simulink model "f16_hifi_euler_vTrim"  (R2020b)
settings: Solver=ode4  StartTime=0.0  StopTime=simTime  FixedStep=stepTime  RelTol=1e-3
undefined symbols (not defined in the file): data, ft, outputs, s
libraries: libAeroLookUpTables x9, aerolibconvert2 x7, lib6DOFUtilityEquations x6, libTFActuatorCalc x5, aerolibtransform2 x1, libEngineAngMomSpecs x1, libAircraftMoISpecs x1, libAircraftWeightandMassSpec x1, libAircraftWingFusalageSpecs x1, libCmdPowConversion x1, libEngineThrustCalc x1, libAtmosphereModel x1
(part 3 of 3)

== system f16_hifi_euler_vTrim/F-16 HiFi Model/Aerodynamic Model/Subsystem/Aerodynamic Forces ==
  note: Wind Axis Forces
  note: Direction Cosine Matrix
  note: Coeffs
  note: Forces
  note: Input Variables
  note: Units
      | Inputs:
      | C_{i}: [ ]
      | qbar: lb/ft^2
      | S: ft^2
      | alpha: deg
      | beta: deg
      | Outputs:
      | F_{i}: lbf
      | M_{i}: lbf*ft
  C_i : Inport
  qbar : Inport  Port=2
  alpha : Inport  Port=3
  beta : Inport  Port=4
  Constant : Constant  Value=S
  Demux : Demux  Outputs=3
  Demux1 : Demux  Outputs=3
  Direction Cosine Matrix Body to Wind : aerolibtransform2/Direction Cosine Matrix Body to Wind
      settings: SourceProductBaseCode=AE
  Gain : Gain  Gain=-1
  Matrix Multiply : Product  Multiplication=Matrix(*)
  Mux : Mux  Inputs=2
  Mux1 : Mux  Inputs=3
  Product : Product  Inputs=3
  Product1 : Product  Inputs=3
  Product2 : Product  Inputs=3
  Fx : Outport  VectorParamsAs1DForOutWhenUnconnected=off
  Fy : Outport  Port=2  VectorParamsAs1DForOutWhenUnconnected=off
  Fz : Outport  Port=3  VectorParamsAs1DForOutWhenUnconnected=off
  D : Outport  Port=4  VectorParamsAs1DForOutWhenUnconnected=off
  C : Outport  Port=5  VectorParamsAs1DForOutWhenUnconnected=off
  L : Outport  Port=6  VectorParamsAs1DForOutWhenUnconnected=off
  wires:
  qbar/1 -> [qbar]
  Constant/1 -> [S]
  Demux/1 -> [Cx]
  Demux/2 -> [Cy]
  Demux/3 -> [Cz]
  [S] -> Product/3
  [qbar] -> Product/2
  [Cz] -> Product/1
  [S] -> Product2/3
  [qbar] -> Product2/2
  [Cx] -> Product2/1
  [Cy] -> Product1/1
  [qbar] -> Product1/2
  [S] -> Product1/3
  Product2/1 -> Fx/1, Mux1/1
  Product1/1 -> Fy/1, Mux1/2
  Product/1 -> Fz/1, Mux1/3
  C_i/1 -> Demux/1
  alpha/1 -> [alpha]
  beta/1 -> [beta]
  [alpha] -> Mux/1
  [beta] -> Mux/2
  Mux/1 -> Direction Cosine Matrix Body to Wind/1
  Direction Cosine Matrix Body to Wind/1 -> Matrix Multiply/1
  Mux1/1 -> Matrix Multiply/2
  Matrix Multiply/1 -> Gain/1
  Gain/1 -> Demux1/1
  Demux1/1 -> D/1
  Demux1/2 -> C/1
  Demux1/3 -> L/1

== system f16_hifi_euler_vTrim/F-16 HiFi Model/Aerodynamic Model/Subsystem/Aerodynamic Moments ==
  note: Moments
  note: Input Variables
  note: Coeffs
  note: Units
      | Inputs:
      | C_{i}: [ ]
      | qbar: lb/ft^2
      | S: ft^2
      | cbar: ft
      | b: ft
      | Outputs:
      | F_{i}: lbf
      | M_{i}: lbf*ft
  C_i : Inport
  qbar : Inport  Port=2
  Constant : Constant  Value=S
  Constant1 : Constant  Value=cbar
  Constant2 : Constant  Value=b
  Demux : Demux  Outputs=3
  Product6 : Product  Inputs=4
  Product7 : Product  Inputs=4
  Product8 : Product  Inputs=4
  Ml : Outport  VectorParamsAs1DForOutWhenUnconnected=off
  Mm : Outport  Port=2  VectorParamsAs1DForOutWhenUnconnected=off
  Mn : Outport  Port=3  VectorParamsAs1DForOutWhenUnconnected=off
  wires:
  [qbar] -> Product7/2
  Constant1/1 -> [cbar]
  [S] -> Product7/3
  [b] -> Product8/4
  [Cm] -> Product7/1
  [Cn] -> Product6/1
  [S] -> Product6/3
  [cbar] -> Product7/4
  Constant2/1 -> [b]
  Constant/1 -> [S]
  [b] -> Product6/4
  [Cl] -> Product8/1
  [qbar] -> Product6/2
  [qbar] -> Product8/2
  Product8/1 -> Ml/1
  Product7/1 -> Mm/1
  qbar/1 -> [qbar]
  [S] -> Product8/3
  Product6/1 -> Mn/1
  C_i/1 -> Demux/1
  Demux/3 -> [Cn]
  Demux/2 -> [Cm]
  Demux/1 -> [Cl]

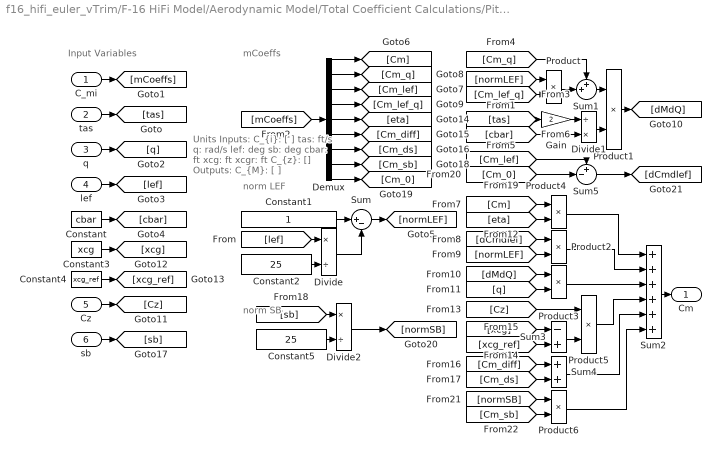
== system f16_hifi_euler_vTrim/F-16 HiFi Model/Aerodynamic Model/Total Coefficient Calculations/Pitch Moment Coefficients ==
  note: norm SB
  note: norm LEF
  note: Input Variables
  note: mCoeffs
  note: Units
      | Inputs:
      | C_{i}: [ ]
      | tas: ft/s
      | q: rad/s
      | lef: deg
      | sb: deg
      | cbar: ft
      | xcg: ft
      | xcgr: ft
      | C_{z}: []
      | Outputs:
      | C_{M}: [ ]
  C_mi : Inport
  tas : Inport  Port=2
  q : Inport  Port=3
  lef : Inport  Port=4
  Cz : Inport  Port=5
  sb : Inport  Port=6
  Constant : Constant  Value=cbar
  Constant1 : Constant
  Constant2 : Constant  Value=25
  Constant3 : Constant  Value=xcg
  Constant4 : Constant  Value=xcg_ref
  Constant5 : Constant  Value=25
  Demux : Demux  Outputs=9
  Divide : Product  Inputs=*/
  Divide1 : Product  Inputs=/*
  Divide2 : Product  Inputs=*/
  Gain : Gain  Gain=2
  Product{,1..6} (7 alike) : Product
  Sum : Sum  Inputs=|+-
  Sum1 : Sum  Inputs=++|
  Sum2 : Sum  Inputs=++++++
  Sum3 : Sum  Inputs=-+
  Sum4 : Sum
  Sum5 : Sum  Inputs=+-|
  Cm : Outport  VectorParamsAs1DForOutWhenUnconnected=off
  wires:
  sb/1 -> [sb]
  [Cm_lef] -> Sum5/1
  [Cm_0] -> Sum5/2
  Product6/1 -> Sum2/6
  [normSB] -> Product6/1
  [Cm_sb] -> Product6/2
  Sum5/1 -> [dCmdlef]
  Divide2/1 -> [normSB]
  [sb] -> Divide2/1
  Constant5/1 -> Divide2/2
  Demux/9 -> [Cm_0]
  Demux/8 -> [Cm_sb]
  Product5/1 -> Sum2/4
  Sum4/1 -> Sum2/5
  [Cm_diff] -> Sum4/1
  [Cm_ds] -> Sum4/2
  Sum3/1 -> Product5/2
  [Cz] -> Product5/1
  [xcg] -> Sum3/1
  [xcg_ref] -> Sum3/2
  Product4/1 -> Sum2/1
  [eta] -> Product4/2
  Demux/5 -> [eta]
  Demux/6 -> [Cm_diff]
  Demux/7 -> [Cm_ds]
  Constant4/1 -> [xcg_ref]
  Constant3/1 -> [xcg]
  Cz/1 -> [Cz]
  tas/1 -> [tas]
  q/1 -> [q]
  Divide/1 -> Sum/2
  C_mi/1 -> [mCoeffs]
  [q] -> Product3/2
  Constant1/1 -> Sum/1
  Constant2/1 -> Divide/2
  Constant/1 -> [cbar]
  lef/1 -> [lef]
  Product/1 -> Sum1/2
  Demux/2 -> [Cm_q]
  [cbar] -> Divide1/2
  [tas] -> Gain/1
  Product3/1 -> Sum2/3
  Sum/1 -> [normLEF]
  [lef] -> Divide/1
  Demux/4 -> [Cm_lef_q]
  Demux/1 -> [Cm]
  [dMdQ] -> Product3/1
  Demux/3 -> [Cm_lef]
  Product1/1 -> [dMdQ]
  [mCoeffs] -> Demux/1
  [normLEF] -> Product/1
  [Cm_lef_q] -> Product/2
  Sum1/1 -> Product1/1
  Gain/1 -> Divide1/1
  Divide1/1 -> Product1/2
  Sum2/1 -> Cm/1
  [Cm_q] -> Sum1/1
  [dCmdlef] -> Product2/1
  [normLEF] -> Product2/2
  [Cm] -> Product4/1
  Product2/1 -> Sum2/2

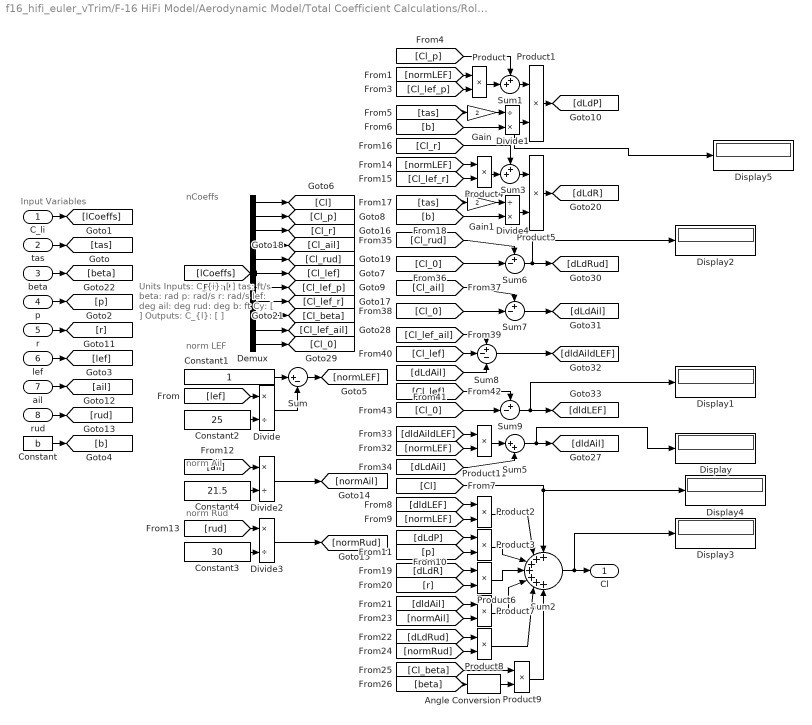
== system f16_hifi_euler_vTrim/F-16 HiFi Model/Aerodynamic Model/Total Coefficient Calculations/Roll Moment Coefficients ==
  note: norm Rud
  note: Input Variables
  note: nCoeffs
  note: norm LEF
  note: norm Ail
  note: Units
      | Inputs:
      | C_{i}: [ ]
      | tas: ft/s
      | beta: rad
      | p: rad/s
      | r: rad/s
      | lef: deg
      | ail: deg
      | rud: deg
      | b: ft
      | Cy: [ ]
      | Outputs:
      | C_{l}: [ ]
  C_li : Inport
  tas : Inport  Port=2
  beta : Inport  Port=3
  p : Inport  Port=4
  r : Inport  Port=5
  lef : Inport  Port=6
  ail : Inport  Port=7
  rud : Inport  Port=8
  Angle Conversion : aerolibconvert2/Angle Conversion  IU=rad  OU=deg
  Constant : Constant  Value=b
  Constant1 : Constant
  Constant2 : Constant  Value=25
  Constant3 : Constant  Value=30
  Constant4 : Constant  Value=21.5
  Demux : Demux  Outputs=11
  Display{,1..5} (6 alike) : Display
  Divide : Product  Inputs=*/
  Divide1 : Product  Inputs=/*
  Divide2 : Product  Inputs=*/
  Divide3 : Product  Inputs=*/
  Divide4 : Product  Inputs=/*
  Gain : Gain  Gain=2
  Gain1 : Gain  Gain=2
  Product{,1..9,11} (11 alike) : Product
  Sum : Sum  Inputs=|+-
  Sum1 : Sum  Inputs=++|
  Sum2 : Sum  Inputs=+++++++
  Sum3 : Sum  Inputs=++|
  Sum5 : Sum  Inputs=|++
  Sum6 : Sum  Inputs=+-|
  Sum7 : Sum  Inputs=+-|
  Sum8 : Sum  Inputs=+--
  Sum9 : Sum  Inputs=+-|
  Cl : Outport  VectorParamsAs1DForOutWhenUnconnected=off
  wires:
  Angle Conversion/1 -> Product9/2
  [beta] -> Angle Conversion/1
  Demux/1 -> [Cl]
  Sum5/1 -> Display/1, [dldAil]
  [normLEF] -> Product2/2
  Product1/1 -> [dLdP]
  tas/1 -> [tas]
  Sum2/1 -> Display3/1, Cl/1
  [dLdRud] -> Product8/1
  [Cl_beta] -> Product9/1
  Demux/3 -> [Cl_r]
  Demux/7 -> [Cl_lef_p]
  [ail] -> Divide2/1
  Product8/1 -> Sum2/6
  Constant4/1 -> Divide2/2
  [normLEF] -> Product4/1
  Constant1/1 -> Sum/1
  Sum1/1 -> Product1/1
  Constant/1 -> [b]
  [normLEF] -> Product11/2
  [Cl] -> Display4/1, Sum2/1
  Sum/1 -> [normLEF]
  [dldAil] -> Product7/1
  Product11/1 -> Sum5/1
  rud/1 -> [rud]
  [Cl_lef_r] -> Product4/2
  [tas] -> Gain1/1
  Demux/4 -> [Cl_ail]
  [dLdP] -> Product3/1
  [p] -> Product3/2
  [dldAildLEF] -> Product11/1
  Divide4/1 -> Product5/2
  [dLdAil] -> Sum5/2
  Sum8/1 -> [dldAildLEF]
  Demux/10 -> [Cl_lef_ail]
  Product5/1 -> [dLdR]
  Product9/1 -> Sum2/7
  C_li/1 -> [lCoeffs]
  [b] -> Divide1/2
  [Cl_lef_p] -> Product/2
  Product/1 -> Sum1/2
  Divide2/1 -> [normAil]
  Demux/9 -> [Cl_beta]
  [lef] -> Divide/1
  [b] -> Divide4/2
  p/1 -> [p]
  [r] -> Product6/2
  [normLEF] -> Product/1
  [rud] -> Divide3/1
  Product3/1 -> Sum2/3
  Gain/1 -> Divide1/1
  Constant2/1 -> Divide/2
  Demux/5 -> [Cl_rud]
  Divide/1 -> Sum/2
  Product7/1 -> Sum2/5
  Sum6/1 -> Display2/1, [dLdRud]
  Demux/2 -> [Cl_p]
  [Cl_p] -> Sum1/1
  Product2/1 -> Sum2/2
  [dLdR] -> Product6/1
  Product6/1 -> Sum2/4
  [tas] -> Gain/1
  [normAil] -> Product7/2
  [Cl_r] -> Sum3/1
  Product4/1 -> Sum3/2
  Divide3/1 -> [normRud]
  ail/1 -> [ail]
  Sum3/1 -> Product5/1
  lef/1 -> [lef]
  Demux/6 -> [Cl_lef]
  Gain1/1 -> Divide4/1
  [Cl_0] -> Sum7/2
  Demux/8 -> [Cl_lef_r]
  [dldLEF] -> Product2/1
  r/1 -> [r]
  beta/1 -> [beta]
  [normRud] -> Product8/2
  Constant3/1 -> Divide3/2
  [lCoeffs] -> Demux/1
  Demux/11 -> [Cl_0]
  [Cl_rud] -> Sum6/1
  [Cl_0] -> Sum6/2
  Sum9/1 -> Display1/1, [dldLEF]
  [Cl_0] -> Sum9/2
  [Cl_lef] -> Sum8/2
  [Cl_ail] -> Sum7/1
  Sum7/1 -> [dLdAil]
  [dLdAil] -> Sum8/3
  [Cl_lef] -> Sum9/1
  [Cl_lef_ail] -> Sum8/1
  Divide1/1 -> Display5/1, Product1/2

== system f16_hifi_euler_vTrim/F-16 HiFi Model/Aerodynamic Model/Total Coefficient Calculations/X-Axis Force Coefficients ==
  note: norm SB
  note: xCoeffs
  note: Input Variables
  note: Units
      | Inputs:
      | C_{i}: [ ]
      | tas: ft/s
      | q: rad/s
      | lef: deg
      | sb: deg
      | cbar: ft
      | Outputs:
      | C_{X}: [ ]
  note: norm LEF
  C_xi : Inport
  tas : Inport  Port=2
  q : Inport  Port=3
  lef : Inport  Port=4
  sb : Inport  Port=5
  Constant : Constant  Value=cbar
  Constant1 : Constant
  Constant2 : Constant  Value=25
  Constant3 : Constant  Value=60
  Demux : Demux  Outputs=6
  Divide : Product  Inputs=*/
  Divide1 : Product  Inputs=/**
  Divide2 : Product  Inputs=*/
  Gain : Gain  Gain=2
  Product{,1..3} (4 alike) : Product
  Sum : Sum  Inputs=|+-
  Sum1 : Sum  Inputs=++|
  Sum2 : Sum  Inputs=++++
  Sum3 : Sum  Inputs=+-|
  Cx : Outport  VectorParamsAs1DForOutWhenUnconnected=off
  wires:
  Product3/1 -> Sum2/4
  [normSB] -> Product3/1
  [Cx_sb] -> Product3/2
  Divide2/1 -> [normSB]
  Constant3/1 -> Divide2/2
  [sb] -> Divide2/1
  Sum3/1 -> [dCxLef]
  [Cx_0] -> Sum3/2
  [Cx_lef] -> Sum3/1
  Demux/6 -> [Cx_0]
  [q] -> Divide1/3
  sb/1 -> [sb]
  Demux/5 -> [Cx_sb]
  Sum2/1 -> Cx/1
  [Cx] -> Sum2/1
  [dXdQ] -> Sum2/3
  Product2/1 -> Sum2/2
  [dCxLef] -> Product2/1
  [normLEF] -> Product2/2
  Product1/1 -> [dXdQ]
  Sum1/1 -> Product1/1
  Divide1/1 -> Product1/2
  [cbar] -> Divide1/2
  Gain/1 -> Divide1/1
  [tas] -> Gain/1
  Product/1 -> Sum1/2
  [Cx_q] -> Sum1/1
  [Cx_lef_q] -> Product/2
  [normLEF] -> Product/1
  Demux/4 -> [Cx_lef_q]
  Demux/3 -> [Cx_lef]
  Demux/2 -> [Cx_q]
  Demux/1 -> [Cx]
  [xCoeffs] -> Demux/1
  Sum/1 -> [normLEF]
  Constant1/1 -> Sum/1
  Divide/1 -> Sum/2
  [lef] -> Divide/1
  Constant2/1 -> Divide/2
  Constant/1 -> [cbar]
  lef/1 -> [lef]
  q/1 -> [q]
  C_xi/1 -> [xCoeffs]
  tas/1 -> [tas]

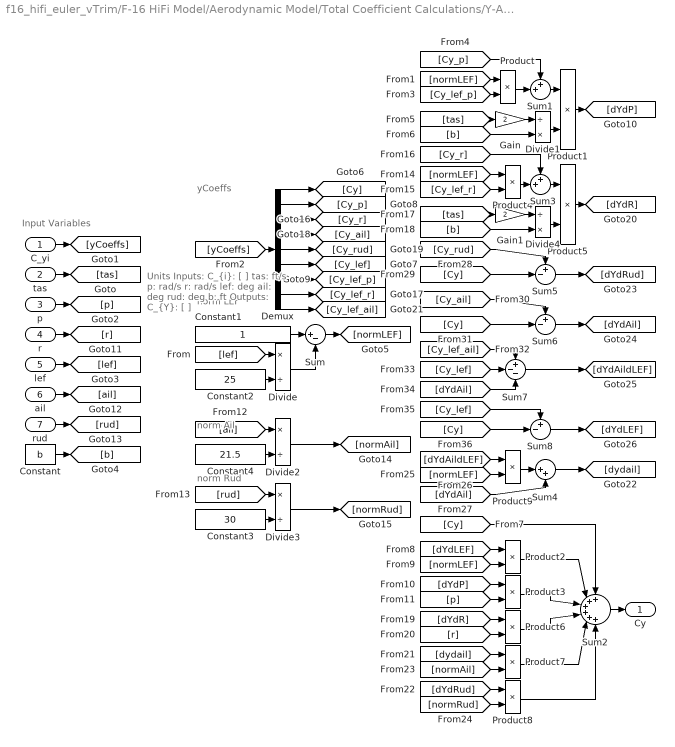
== system f16_hifi_euler_vTrim/F-16 HiFi Model/Aerodynamic Model/Total Coefficient Calculations/Y-Axis Force Coefficients ==
  note: norm Rud
  note: norm Ail
  note: norm LEF
  note: Input Variables
  note: yCoeffs
  note: Units
      | Inputs:
      | C_{i}: [ ]
      | tas: ft/s
      | p: rad/s
      | r: rad/s
      | lef: deg
      | ail: deg
      | rud: deg
      | b: ft
      | Outputs:
      | C_{Y}: [ ]
  C_yi : Inport
  tas : Inport  Port=2
  p : Inport  Port=3
  r : Inport  Port=4
  lef : Inport  Port=5
  ail : Inport  Port=6
  rud : Inport  Port=7
  Constant : Constant  Value=b
  Constant1 : Constant
  Constant2 : Constant  Value=25
  Constant3 : Constant  Value=30
  Constant4 : Constant  Value=21.5
  Demux : Demux  Outputs=9
  Divide : Product  Inputs=*/
  Divide1 : Product  Inputs=/*
  Divide2 : Product  Inputs=*/
  Divide3 : Product  Inputs=*/
  Divide4 : Product  Inputs=/*
  Gain : Gain  Gain=2
  Gain1 : Gain  Gain=2
  Product{,1..9} (10 alike) : Product
  Sum : Sum  Inputs=|+-
  Sum1 : Sum  Inputs=++|
  Sum2 : Sum  Inputs=++++++
  Sum3 : Sum  Inputs=++|
  Sum4 : Sum  Inputs=|++
  Sum5 : Sum  Inputs=+-|
  Sum6 : Sum  Inputs=+-|
  Sum7 : Sum  Inputs=+--
  Sum8 : Sum  Inputs=+-|
  Cy : Outport  VectorParamsAs1DForOutWhenUnconnected=off
  wires:
  [Cy_lef] -> Sum8/1
  [Cy] -> Sum8/2
  Sum8/1 -> [dYdLEF]
  Sum7/1 -> [dYdAildLEF]
  [Cy_lef] -> Sum7/2
  [dYdAil] -> Sum7/3
  [Cy_lef_ail] -> Sum7/1
  [Cy_ail] -> Sum6/1
  Sum6/1 -> [dYdAil]
  [Cy] -> Sum6/2
  Sum5/1 -> [dYdRud]
  [Cy] -> Sum5/2
  [Cy_rud] -> Sum5/1
  Sum4/1 -> [dydail]
  [dYdAil] -> Sum4/2
  Product9/1 -> Sum4/1
  [dYdAildLEF] -> Product9/1
  [normLEF] -> Product9/2
  Demux/9 -> [Cy_lef_ail]
  Product7/1 -> Sum2/5
  Product8/1 -> Sum2/6
  [Cy] -> Sum2/1
  Product2/1 -> Sum2/2
  Product3/1 -> Sum2/3
  Product6/1 -> Sum2/4
  Sum2/1 -> Cy/1
  [dydail] -> Product7/1
  [normAil] -> Product7/2
  [dYdRud] -> Product8/1
  [normRud] -> Product8/2
  [dYdR] -> Product6/1
  [r] -> Product6/2
  Product5/1 -> [dYdR]
  Product4/1 -> Sum3/2
  Gain1/1 -> Divide4/1
  [Cy_r] -> Sum3/1
  [tas] -> Gain1/1
  Sum3/1 -> Product5/1
  [Cy_lef_r] -> Product4/2
  Divide4/1 -> Product5/2
  [normLEF] -> Product4/1
  [b] -> Divide4/2
  Demux/4 -> [Cy_ail]
  Demux/5 -> [Cy_rud]
  Demux/8 -> [Cy_lef_r]
  Demux/3 -> [Cy_r]
  [rud] -> Divide3/1
  Constant3/1 -> Divide3/2
  Divide3/1 -> [normRud]
  Constant4/1 -> Divide2/2
  [ail] -> Divide2/1
  Divide2/1 -> [normAil]
  rud/1 -> [rud]
  ail/1 -> [ail]
  r/1 -> [r]
  Constant1/1 -> Sum/1
  [p] -> Product3/2
  Demux/6 -> [Cy_lef]
  [dYdP] -> Product3/1
  [tas] -> Gain/1
  [Cy_p] -> Sum1/1
  Product/1 -> Sum1/2
  Divide/1 -> Sum/2
  p/1 -> [p]
  Demux/7 -> [Cy_lef_p]
  [lef] -> Divide/1
  tas/1 -> [tas]
  Sum/1 -> [normLEF]
  Constant/1 -> [b]
  [normLEF] -> Product/1
  Product1/1 -> [dYdP]
  [yCoeffs] -> Demux/1
  [b] -> Divide1/2
  C_yi/1 -> [yCoeffs]
  [normLEF] -> Product2/2
  Divide1/1 -> Product1/2
  Gain/1 -> Divide1/1
  Constant2/1 -> Divide/2
  [Cy_lef_p] -> Product/2
  Sum1/1 -> Product1/1
  [dYdLEF] -> Product2/1
  lef/1 -> [lef]
  Demux/1 -> [Cy]
  Demux/2 -> [Cy_p]

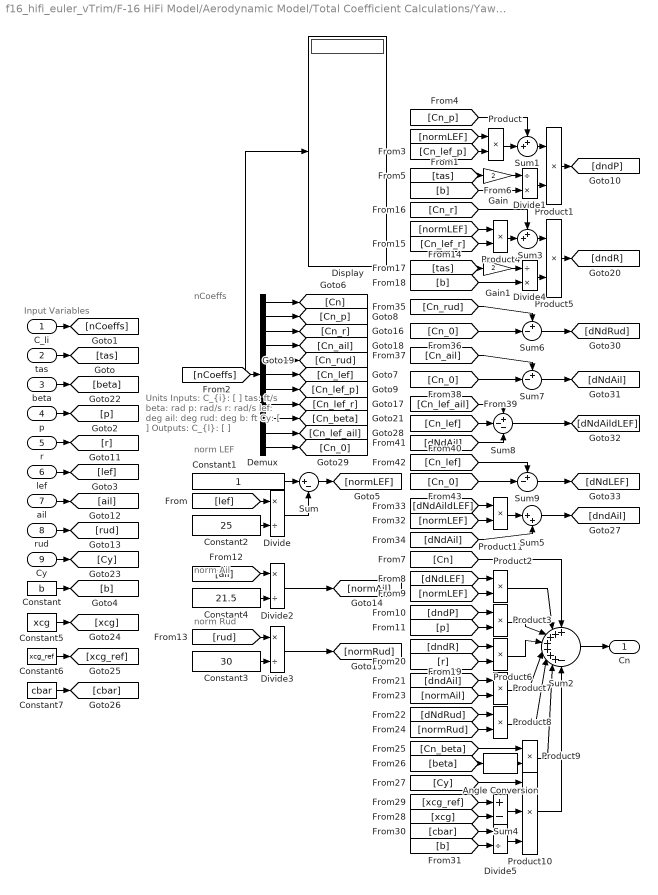
== system f16_hifi_euler_vTrim/F-16 HiFi Model/Aerodynamic Model/Total Coefficient Calculations/Yaw Moment Coefficients ==
  note: norm Rud
  note: norm Ail
  note: norm LEF
  note: Units
      | Inputs:
      | C_{i}: [ ]
      | tas: ft/s
      | beta: rad
      | p: rad/s
      | r: rad/s
      | lef: deg
      | ail: deg
      | rud: deg
      | b: ft
      | Cy: [ ]
      | Outputs:
      | C_{l}: [ ]
  note: nCoeffs
  note: Input Variables
  C_li : Inport
  tas : Inport  Port=2
  beta : Inport  Port=3
  p : Inport  Port=4
  r : Inport  Port=5
  lef : Inport  Port=6
  ail : Inport  Port=7
  rud : Inport  Port=8
  Cy : Inport  Port=9
  Angle Conversion : aerolibconvert2/Angle Conversion  IU=rad  OU=deg
  Constant : Constant  Value=b
  Constant1 : Constant
  Constant2 : Constant  Value=25
  Constant3 : Constant  Value=30
  Constant4 : Constant  Value=21.5
  Constant5 : Constant  Value=xcg
  Constant6 : Constant  Value=xcg_ref
  Constant7 : Constant  Value=cbar
  Demux : Demux  Outputs=11
  Display : Display
  Divide{,2..3,5} (4 alike) : Product  Inputs=*/
  Divide1 : Product  Inputs=/*
  Divide4 : Product  Inputs=/*
  Gain : Gain  Gain=2
  Gain1 : Gain  Gain=2
  Product{,1..9,11} (11 alike) : Product
  Product10 : Product  Inputs=3
  Sum : Sum  Inputs=|+-
  Sum1 : Sum  Inputs=++|
  Sum2 : Sum  Inputs=+++++++-
  Sum3 : Sum  Inputs=++|
  Sum4 : Sum  Inputs=+-
  Sum5 : Sum  Inputs=|++
  Sum6 : Sum  Inputs=+-|
  Sum7 : Sum  Inputs=+-|
  Sum8 : Sum  Inputs=+--
  Sum9 : Sum  Inputs=+-|
  Cn : Outport  VectorParamsAs1DForOutWhenUnconnected=off
  wires:
  Angle Conversion/1 -> Product9/2
  [beta] -> Angle Conversion/1
  [Cn_lef] -> Sum9/1
  [Cn_lef_ail] -> Sum8/1
  [dNdAil] -> Sum8/3
  [Cn_ail] -> Sum7/1
  Sum7/1 -> [dNdAil]
  [Cn_0] -> Sum9/2
  [Cn_lef] -> Sum8/2
  [Cn_0] -> Sum7/2
  [Cn_0] -> Sum6/2
  Sum9/1 -> [dNdLEF]
  [Cn_rud] -> Sum6/1
  Sum8/1 -> [dNdAildLEF]
  Demux/11 -> [Cn_0]
  Demux/10 -> [Cn_lef_ail]
  [dNdAildLEF] -> Product11/1
  Product11/1 -> Sum5/1
  [normLEF] -> Product11/2
  Sum5/1 -> [dndAil]
  [dNdAil] -> Sum5/2
  Product10/1 -> Sum2/8
  [Cy] -> Product10/1
  Divide5/1 -> Product10/3
  Sum4/1 -> Product10/2
  [b] -> Divide5/2
  [cbar] -> Divide5/1
  [xcg] -> Sum4/2
  [xcg_ref] -> Sum4/1
  Constant7/1 -> [cbar]
  Constant5/1 -> [xcg]
  Constant6/1 -> [xcg_ref]
  Cy/1 -> [Cy]
  [Cn_beta] -> Product9/1
  r/1 -> [r]
  Sum/1 -> [normLEF]
  Sum2/1 -> Cn/1
  lef/1 -> [lef]
  Demux/6 -> [Cn_lef]
  rud/1 -> [rud]
  ail/1 -> [ail]
  beta/1 -> [beta]
  [normRud] -> Product8/2
  [Cn_lef_r] -> Product4/2
  Gain1/1 -> Divide4/1
  Constant3/1 -> Divide3/2
  Demux/1 -> [Cn]
  Product6/1 -> Sum2/4
  Demux/5 -> [Cn_rud]
  Product7/1 -> Sum2/5
  Divide3/1 -> [normRud]
  [dndR] -> Product6/1
  Product8/1 -> Sum2/6
  Product4/1 -> Sum3/2
  Demux/8 -> [Cn_lef_r]
  Demux/7 -> [Cn_lef_p]
  Constant4/1 -> Divide2/2
  [Cn_r] -> Sum3/1
  Demux/2 -> [Cn_p]
  Gain/1 -> Divide1/1
  Divide/1 -> Sum/2
  [ail] -> Divide2/1
  [Cn_p] -> Sum1/1
  Product2/1 -> Sum2/2
  [tas] -> Gain/1
  Product3/1 -> Sum2/3
  [p] -> Product3/2
  Sum3/1 -> Product5/1
  Constant1/1 -> Sum/1
  Constant2/1 -> Divide/2
  [normLEF] -> Product4/1
  [dNdRud] -> Product8/1
  [rud] -> Divide3/1
  Demux/4 -> [Cn_ail]
  [b] -> Divide4/2
  [normLEF] -> Product/1
  p/1 -> [p]
  [lef] -> Divide/1
  tas/1 -> [tas]
  Divide2/1 -> [normAil]
  [r] -> Product6/2
  Sum1/1 -> Product1/1
  Product/1 -> Sum1/2
  Divide1/1 -> Product1/2
  Demux/3 -> [Cn_r]
  [Cn] -> Sum2/1
  Constant/1 -> [b]
  Divide4/1 -> Product5/2
  [Cn_lef_p] -> Product/2
  [dNdLEF] -> Product2/1
  [b] -> Divide1/2
  [normAil] -> Product7/2
  [dndP] -> Product3/1
  [dndAil] -> Product7/1
  [tas] -> Gain1/1
  [normLEF] -> Product2/2
  C_li/1 -> [nCoeffs]
  Product9/1 -> Sum2/7
  Demux/9 -> [Cn_beta]
  Product1/1 -> [dndP]
  Product5/1 -> [dndR]
  Sum6/1 -> [dNdRud]
  [nCoeffs] -> Display/1, Demux/1

== system f16_hifi_euler_vTrim/F-16 HiFi Model/Aerodynamic Model/Total Coefficient Calculations/Z-Axis Force Coefficients ==
  note: xCoeffs
  note: Units
      | Inputs:
      | C_{i}: [ ]
      | tas: ft/s
      | q: rad/s
      | lef: deg
      | sb: deg
      | cbar: ft
      | Outputs:
      | C_{X}: [ ]
  note: norm LEF
  note: Input Variables
  note: norm SB
  C_zi : Inport
  tas : Inport  Port=2
  q : Inport  Port=3
  lef : Inport  Port=4
  sb : Inport  Port=5
  Constant : Constant  Value=cbar
  Constant1 : Constant
  Constant2 : Constant  Value=25
  Constant3 : Constant  Value=25
  Demux : Demux  Outputs=6
  Divide : Product  Inputs=*/
  Divide1 : Product  Inputs=/**
  Divide2 : Product  Inputs=*/
  Gain : Gain  Gain=2
  Product{,1..3} (4 alike) : Product
  Sum : Sum  Inputs=|+-
  Sum1 : Sum  Inputs=++|
  Sum2 : Sum  Inputs=++++
  Sum3 : Sum  Inputs=+-|
  Cz : Outport  VectorParamsAs1DForOutWhenUnconnected=off
  wires:
  tas/1 -> [tas]
  Divide/1 -> Sum/2
  Demux/3 -> [Cz_lef]
  Divide2/1 -> [normSB]
  [Cz] -> Sum2/1
  [normLEF] -> Product2/2
  Product1/1 -> [dZdQ]
  Sum1/1 -> Product1/1
  lef/1 -> [lef]
  Product2/1 -> Sum2/2
  Sum/1 -> [normLEF]
  Sum2/1 -> Cz/1
  [tas] -> Gain/1
  Demux/6 -> [Cz_0]
  Gain/1 -> Divide1/1
  [cbar] -> Divide1/2
  [zCoeffs] -> Demux/1
  [Cz_lef] -> Sum3/1
  [q] -> Divide1/3
  Product/1 -> Sum1/2
  Demux/2 -> [Cz_q]
  Constant2/1 -> Divide/2
  C_zi/1 -> [zCoeffs]
  [lef] -> Divide/1
  sb/1 -> [sb]
  Sum3/1 -> [dCzLef]
  Constant1/1 -> Sum/1
  Constant/1 -> [cbar]
  q/1 -> [q]
  Divide1/1 -> Product1/2
  Demux/1 -> [Cz]
  [dCzLef] -> Product2/1
  Demux/4 -> [Cz_lef_q]
  [sb] -> Divide2/1
  [normLEF] -> Product/1
  [Cz_lef_q] -> Product/2
  [Cz_q] -> Sum1/1
  [normSB] -> Product3/1
  Constant3/1 -> Divide2/2
  [Cz_sb] -> Product3/2
  [dZdQ] -> Sum2/3
  [Cz_0] -> Sum3/2
  Demux/5 -> [Cz_sb]
  Product3/1 -> Sum2/4

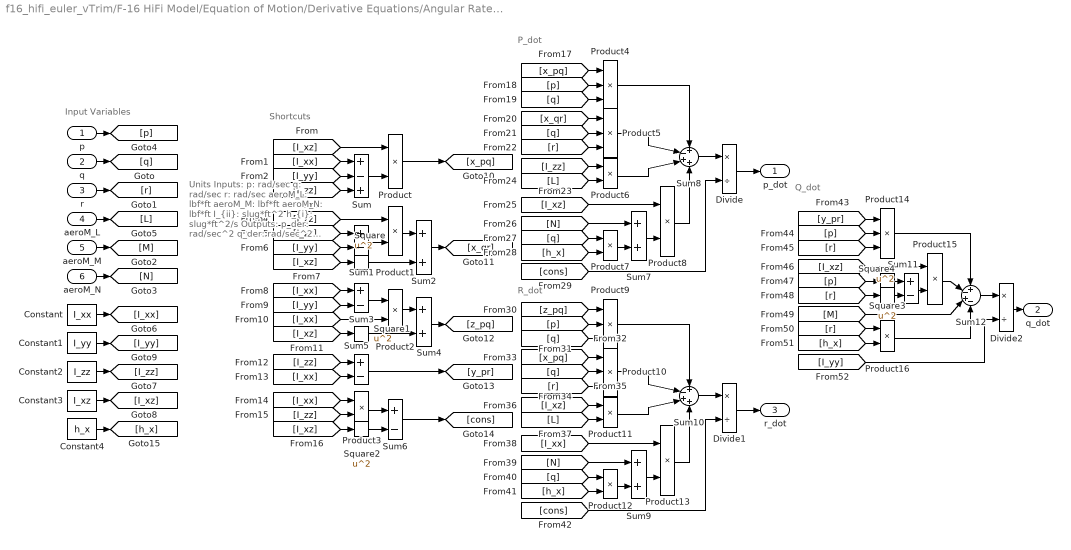
== system f16_hifi_euler_vTrim/F-16 HiFi Model/Equation of Motion/Derivative Equations/Angular Rate Equations ==
  note: Q_dot
  note: P_dot
  note: Shortcuts
  note: Units
      | Inputs:
      | p: rad/sec
      | q: rad/sec
      | r: rad/sec
      | aeroM_L: lbf*ft
      | aeroM_M: lbf*ft
      | aeroM_N: lbf*ft
      | I_{ii}: slug*ft^2
      | h_{i}: slug*ft^2/s
      | Outputs:
      | p_der: rad/sec^2
      | q_der: rad/sec^2
      | r_der: rad/sec^2
  note: Input Variables
  note: R_dot
  p : Inport
  q : Inport  Port=2
  r : Inport  Port=3
  aeroM_L : Inport  Port=4
  aeroM_M : Inport  Port=5
  aeroM_N : Inport  Port=6
  Constant : Constant  Value=I_xx
  Constant1 : Constant  Value=I_yy
  Constant2 : Constant  Value=I_zz
  Constant3 : Constant  Value=I_xz
  Constant4 : Constant  Value=h_x
  Divide : Product  Inputs=*/
  Divide1 : Product  Inputs=*/
  Divide2 : Product  Inputs=*/
  Product{,1..3,6..8,11..13,15..16} (12 alike) : Product
  Product{4..5,9..10,14} (5 alike) : Product  Inputs=3
  Square{,1..4} (5 alike) : Math  Operator=square  SignedPower=on  SaturateOnIntegerOverflow=on
  Sum : Sum  Inputs=+-+
  Sum{1,3,5..6,11} (5 alike) : Sum  Inputs=+-
  Sum10 : Sum  Inputs=+-++
  Sum12 : Sum  Inputs=+-+-
  Sum{2,4,7,9} (4 alike) : Sum
  Sum8 : Sum  Inputs=+-++
  p_dot : Outport  VectorParamsAs1DForOutWhenUnconnected=off
  q_dot : Outport  Port=2  VectorParamsAs1DForOutWhenUnconnected=off
  r_dot : Outport  Port=3  VectorParamsAs1DForOutWhenUnconnected=off
  wires:
  p/1 -> [p]
  q/1 -> [q]
  r/1 -> [r]
  aeroM_L/1 -> [L]
  aeroM_M/1 -> [M]
  aeroM_N/1 -> [N]
  Constant/1 -> [I_xx]
  Constant3/1 -> [I_xz]
  Constant2/1 -> [I_zz]
  Constant1/1 -> [I_yy]
  [I_xx] -> Sum/1
  [I_zz] -> Sum/3
  [I_yy] -> Sum/2
  [I_xz] -> Product/1
  Sum/1 -> Product/2
  Product/1 -> [x_pq]
  [I_xz] -> Square/1
  [I_zz] -> Sum1/1
  [I_yy] -> Sum1/2
  Sum1/1 -> Product1/2
  [I_zz] -> Product1/1
  Product1/1 -> Sum2/1
  Square/1 -> Sum2/2
  Sum2/1 -> [x_qr]
  [I_xz] -> Square1/1
  [I_xx] -> Product2/2
  [I_yy] -> Sum3/2
  [I_xx] -> Sum3/1
  Sum3/1 -> Product2/1
  Product2/1 -> Sum4/1
  Square1/1 -> Sum4/2
  Sum4/1 -> [z_pq]
  [I_zz] -> Sum5/1
  [I_xx] -> Sum5/2
  Sum5/1 -> [y_pr]
  [I_zz] -> Product3/2
  [I_xx] -> Product3/1
  [I_xz] -> Square2/1
  Product3/1 -> Sum6/1
  Square2/1 -> Sum6/2
  Sum6/1 -> [cons]
  Constant4/1 -> [h_x]
  [x_pq] -> Product4/1
  [p] -> Product4/2
  [q] -> Product4/3
  [q] -> Product5/2
  [x_qr] -> Product5/1
  [r] -> Product5/3
  [I_zz] -> Product6/1
  [L] -> Product6/2
  [q] -> Product7/1
  [h_x] -> Product7/2
  [N] -> Sum7/1
  [I_xz] -> Product8/1
  Product7/1 -> Sum7/2
  Sum7/1 -> Product8/2
  Product6/1 -> Sum8/3
  Product5/1 -> Sum8/2
  Product4/1 -> Sum8/1
  Product8/1 -> Sum8/4
  Sum8/1 -> Divide/1
  Divide/1 -> p_dot/1
  [cons] -> Divide/2
  Product12/1 -> Sum9/2
  Sum9/1 -> Product13/2
  [N] -> Sum9/1
  Sum10/1 -> Divide1/1
  [q] -> Product12/1
  Product13/1 -> Sum10/4
  Product9/1 -> Sum10/1
  [I_xz] -> Product11/1
  [h_x] -> Product12/2
  Divide1/1 -> r_dot/1
  [x_pq] -> Product10/1
  [q] -> Product10/2
  [I_xx] -> Product13/1
  [z_pq] -> Product9/1
  [q] -> Product9/3
  [L] -> Product11/2
  Product10/1 -> Sum10/2
  [p] -> Product9/2
  [cons] -> Divide1/2
  [r] -> Product10/3
  Product11/1 -> Sum10/3
  [y_pr] -> Product14/1
  [p] -> Product14/2
  Product14/1 -> Sum12/1
  [r] -> Product14/3
  [p] -> Square3/1
  [r] -> Square4/1
  Square3/1 -> Sum11/1
  Square4/1 -> Sum11/2
  [I_xz] -> Product15/1
  Sum11/1 -> Product15/2
  [r] -> Product16/1
  [h_x] -> Product16/2
  [M] -> Sum12/3
  Product15/1 -> Sum12/2
  Product16/1 -> Sum12/4
  Sum12/1 -> Divide2/1
  [I_yy] -> Divide2/2
  Divide2/1 -> q_dot/1

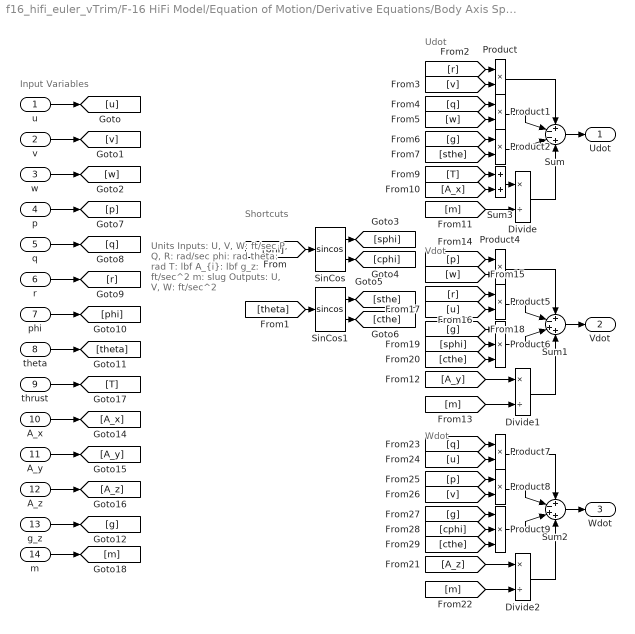
== system f16_hifi_euler_vTrim/F-16 HiFi Model/Equation of Motion/Derivative Equations/Body Axis Speed Equations ==
  note: Vdot
  note: Input Variables
  note: Wdot
  note: Udot
  note: Shortcuts
  note: Units
      | Inputs:
      | U, V, W: ft/sec
      | P, Q, R: rad/sec
      | phi: rad
      | theta: rad
      | T: lbf
      | A_{i}: lbf
      | g_z: ft/sec^2
      | m: slug
      | Outputs:
      | U, V, W: ft/sec^2
  u : Inport
  v : Inport  Port=2
  w : Inport  Port=3
  p : Inport  Port=4
  q : Inport  Port=5
  r : Inport  Port=6
  phi : Inport  Port=7
  theta : Inport  Port=8
  thrust : Inport  Port=9
  A_x : Inport  Port=10
  A_y : Inport  Port=11
  A_z : Inport  Port=12
  g_z : Inport  Port=13
  m : Inport  Port=14
  Divide : Product  Inputs=*/
  Divide1 : Product  Inputs=*/
  Divide2 : Product  Inputs=*/
  Product{,1..2,4..5,7..8} (7 alike) : Product
  Product6 : Product  Inputs=3
  Product9 : Product  Inputs=3
  SinCos : Trigonometry  Operator=sincos
  SinCos1 : Trigonometry  Operator=sincos
  Sum : Sum  Inputs=+--+
  Sum1 : Sum  Inputs=+-++
  Sum2 : Sum  Inputs=+-++
  Sum3 : Sum
  Udot : Outport  VectorParamsAs1DForOutWhenUnconnected=off
  Vdot : Outport  Port=2  VectorParamsAs1DForOutWhenUnconnected=off
  Wdot : Outport  Port=3  VectorParamsAs1DForOutWhenUnconnected=off
  wires:
  u/1 -> [u]
  SinCos/1 -> [sphi]
  v/1 -> [v]
  [phi] -> SinCos/1
  SinCos1/1 -> [sthe]
  SinCos/2 -> [cphi]
  SinCos1/2 -> [cthe]
  [theta] -> SinCos1/1
  [r] -> Product/1
  [v] -> Product/2
  w/1 -> [w]
  p/1 -> [p]
  r/1 -> [r]
  q/1 -> [q]
  theta/1 -> [theta]
  phi/1 -> [phi]
  [w] -> Product1/2
  [q] -> Product1/1
  g_z/1 -> [g]
  [sthe] -> Product2/2
  [g] -> Product2/1
  A_x/1 -> [A_x]
  thrust/1 -> [T]
  [A_x] -> Sum3/2
  [T] -> Sum3/1
  m/1 -> [m]
  Sum/1 -> Udot/1
  Sum3/1 -> Divide/1
  [m] -> Divide/2
  Divide/1 -> Sum/4
  Product1/1 -> Sum/2
  Product/1 -> Sum/1
  [w] -> Product4/2
  [p] -> Product4/1
  [g] -> Product6/1
  [A_y] -> Divide1/1
  Sum1/1 -> Vdot/1
  Product4/1 -> Sum1/1
  [m] -> Divide1/2
  Product6/1 -> Sum1/3
  Product5/1 -> Sum1/2
  [r] -> Product5/1
  [u] -> Product5/2
  Divide1/1 -> Sum1/4
  [sphi] -> Product6/2
  [cthe] -> Product6/3
  [A_z] -> Divide2/1
  Divide2/1 -> Sum2/4
  [p] -> Product8/1
  [cphi] -> Product9/2
  Product9/1 -> Sum2/3
  [q] -> Product7/1
  [m] -> Divide2/2
  Product8/1 -> Sum2/2
  [g] -> Product9/1
  [v] -> Product8/2
  [u] -> Product7/2
  Product7/1 -> Sum2/1
  [cthe] -> Product9/3
  Sum2/1 -> Wdot/1
  A_y/1 -> [A_y]
  A_z/1 -> [A_z]
  Product2/1 -> Sum/3

== system f16_hifi_euler_vTrim/F-16 HiFi Model/Equation of Motion/Derivative Equations/Kinematic Equations ==
  note: Theta_dot
  note: Units
      | Inputs:
      | phi: rad
      | theta: rad
      | p: rad/sec
      | q: rad/sec
      | r: rad/sec
      | Outputs:
      | phi_dot: rad/sec
      | theta_dot: rad/sec
      | psi_dot: rad/sec
  note: Input Variables
  note: Shortcuts
  note: Phi_dot
  note: Psi_dot
  "phi " : Inport
  theta : Inport  Port=2
  p : Inport  Port=3
  q : Inport  Port=4
  r : Inport  Port=5
  Divide : Product  Inputs=*/
  Product{,1..6} (7 alike) : Product
  SinCos : Trigonometry  Operator=sincos
  SinCos1 : Trigonometry  Operator=cos
  SinCos2 : Trigonometry  Operator=tan
  Sum : Sum  Inputs=+-
  Sum1 : Sum  Inputs=|++
  Sum2 : Sum  Inputs=++|
  Sum3 : Sum  Inputs=++|
  phi_dot : Outport  VectorParamsAs1DForOutWhenUnconnected=off
  theta_dot : Outport  Port=2  VectorParamsAs1DForOutWhenUnconnected=off
  psi_dot : Outport  Port=3  VectorParamsAs1DForOutWhenUnconnected=off
  wires:
  "phi "/1 -> [phi]
  p/1 -> [p]
  theta/1 -> [theta]
  q/1 -> [q]
  r/1 -> [r]
  SinCos2/1 -> [tthe]
  SinCos1/1 -> [cthe]
  SinCos/1 -> [sphi]
  SinCos/2 -> [cphi]
  [phi] -> SinCos/1
  [theta] -> SinCos1/1, SinCos2/1
  [q] -> Product/1
  [cphi] -> Product/2
  [sphi] -> Product1/1
  [r] -> Product1/2
  Product/1 -> Sum/1
  Product1/1 -> Sum/2
  Sum/1 -> theta_dot/1
  [q] -> Product2/1
  [sphi] -> Product2/2
  [tthe] -> Product6/1
  [cphi] -> Product3/2
  [r] -> Product3/1
  Product2/1 -> Sum1/1
  [p] -> Sum3/1
  Product3/1 -> Sum1/2
  Sum3/1 -> phi_dot/1
  [cphi] -> Product5/2
  [r] -> Product5/1
  [q] -> Product4/1
  [sphi] -> Product4/2
  Product5/1 -> Sum2/2
  Product4/1 -> Sum2/1
  Sum2/1 -> Divide/1
  [cthe] -> Divide/2
  Divide/1 -> psi_dot/1
  Sum1/1 -> Product6/2
  Product6/1 -> Sum3/2

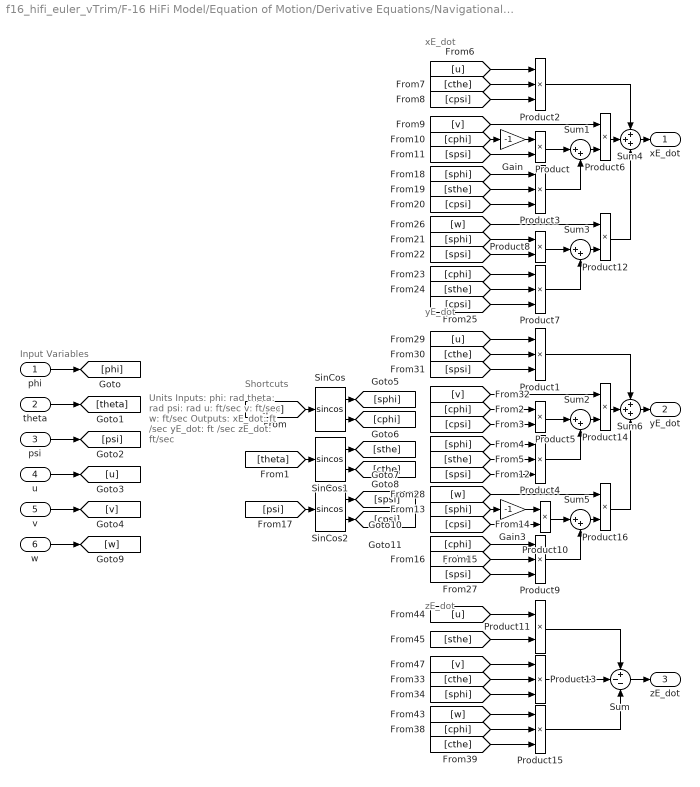
== system f16_hifi_euler_vTrim/F-16 HiFi Model/Equation of Motion/Derivative Equations/Navigational Equations ==
  note: xE_dot
  note: Shortcuts
  note: Input Variables
  note: Units
      | Inputs:
      | phi: rad
      | theta: rad
      | psi: rad
      | u: ft/sec
      | v: ft/sec
      | w: ft/sec
      | Outputs:
      | xE_dot: ft /sec
      | yE_dot: ft /sec
      | zE_dot: ft/sec
  note: yE_dot
  note: zE_dot
  "phi " : Inport
  theta : Inport  Port=2
  psi : Inport  Port=3
  u : Inport  Port=4
  v : Inport  Port=5
  w : Inport  Port=6
  Gain : Gain  Gain=-1
  Gain3 : Gain  Gain=-1
  Product{,5..6,8,10..12,14,16} (9 alike) : Product
  Product{1..4,7,9,13,15} (8 alike) : Product  Inputs=3
  SinCos : Trigonometry  Operator=sincos
  SinCos1 : Trigonometry  Operator=sincos
  SinCos2 : Trigonometry  Operator=sincos
  Sum : Sum  Inputs=+--
  Sum{1..3,5} (4 alike) : Sum  Inputs=|++
  Sum4 : Sum  Inputs=+++
  Sum6 : Sum  Inputs=+++
  xE_dot : Outport  VectorParamsAs1DForOutWhenUnconnected=off
  yE_dot : Outport  Port=2  VectorParamsAs1DForOutWhenUnconnected=off
  zE_dot : Outport  Port=3  VectorParamsAs1DForOutWhenUnconnected=off
  wires:
  v/1 -> [v]
  theta/1 -> [theta]
  "phi "/1 -> [phi]
  [phi] -> SinCos/1
  SinCos/2 -> [cphi]
  u/1 -> [u]
  psi/1 -> [psi]
  SinCos/1 -> [sphi]
  w/1 -> [w]
  SinCos1/2 -> [cthe]
  [theta] -> SinCos1/1
  [psi] -> SinCos2/1
  SinCos2/2 -> [cpsi]
  SinCos2/1 -> [spsi]
  SinCos1/1 -> [sthe]
  [u] -> Product2/1
  [cthe] -> Product2/2
  [cpsi] -> Product2/3
  [cphi] -> Gain/1
  [sthe] -> Product3/2
  [cpsi] -> Product3/3
  [sphi] -> Product3/1
  [spsi] -> Product/2
  [v] -> Product6/1
  Gain/1 -> Product/1
  Product/1 -> Sum1/1
  Product3/1 -> Sum1/2
  [spsi] -> Product8/2
  [w] -> Product12/1
  Product7/1 -> Sum3/2
  [cphi] -> Product7/1
  [cpsi] -> Product7/3
  [sthe] -> Product7/2
  [sphi] -> Product8/1
  Product8/1 -> Sum3/1
  Product2/1 -> Sum4/1
  Sum1/1 -> Product6/2
  Sum4/1 -> xE_dot/1
  Product9/1 -> Sum5/2
  Product1/1 -> Sum6/1
  Sum6/1 -> yE_dot/1
  [u] -> Product1/1
  [cthe] -> Product1/2
  [spsi] -> Product1/3
  [sthe] -> Product4/2
  Gain3/1 -> Product10/1
  Product5/1 -> Sum2/1
  Product10/1 -> Sum5/1
  [cphi] -> Product5/1
  [spsi] -> Product9/3
  [cpsi] -> Product10/2
  [w] -> Product16/1
  [sthe] -> Product9/2
  [sphi] -> Gain3/1
  Product4/1 -> Sum2/2
  [cphi] -> Product9/1
  [cpsi] -> Product5/2
  [sphi] -> Product4/1
  [spsi] -> Product4/3
  [v] -> Product13/1
  [u] -> Product11/1
  [sthe] -> Product11/2
  [cphi] -> Product15/2
  [cthe] -> Product13/2
  [cthe] -> Product15/3
  [w] -> Product15/1
  [sphi] -> Product13/3
  Product11/1 -> Sum/1
  Product13/1 -> Sum/2
  Product15/1 -> Sum/3
  Sum/1 -> zE_dot/1
  Product6/1 -> Sum4/2
  Sum3/1 -> Product12/2
  Product12/1 -> Sum4/3
  Sum2/1 -> Product14/2
  Product14/1 -> Sum6/2
  [v] -> Product14/1
  Sum5/1 -> Product16/2
  Product16/1 -> Sum6/3

== system f16_hifi_euler_vTrim/F-16 HiFi Model/Equation of Motion/Derivative Equations/Power Rate ==
  note: Power Rate Calc
  note: Input Variables
  note: Units
      | Inputs:
      | cmdPower: Hp
      | actPower: Hp
      | Outputs:
      | Power: Hp
  note: If Condition
  note: If
  note: Else
  commanded Power : Inport
  Power : Inport  Port=2
  If : If  IfExpression=u1 >= 50
  Merge : Merge
  Merge1 : Merge
  Product : Product
  Sum : Sum  Inputs=-+
  cmd If : Subsystem  TreatAsAtomicUnit=on
  cmd else : Subsystem  TreatAsAtomicUnit=on
  powerDot : Outport  VectorParamsAs1DForOutWhenUnconnected=off
  wires:
  commanded Power/1 -> [cmdPower]
  [cmdPower] -> If/1
  If/1 -> [if]
  If/2 -> [else]
  [if] -> cmd If/Action
  [else] -> cmd else/Action
  Merge/1 -> [T]
  Merge1/1 -> [P2]
  [power] -> Sum/1
  [P2] -> Sum/2
  Sum/1 -> Product/2
  [T] -> Product/1
  Product/1 -> powerDot/1
  [power] -> cmd If/2(Power)
  [cmdPower] -> cmd If/1(cmdPower)
  [power] -> cmd else/2(Power)
  [cmdPower] -> cmd else/1(cmdPower)
  cmd else/2(P2) -> Merge1/2
  cmd If/1(T) -> Merge/1
  cmd If/2(P2) -> Merge1/1
  cmd else/1(T) -> Merge/2
  Power/1 -> [power]

== system f16_hifi_euler_vTrim/F-16 HiFi Model/Equation of Motion/Derivative Equations/Wind Axis Param Equations ==
  note: Units
      | Inputs:
      | tas: ft/sec
      | alpha: rad
      | U, V, W: ft/sec
      | U, V, Wdot: ft/sec^2
      | Outputs:
      | tas_dot: ft/sec^2
      | alpha_dot: rad/sec
      | beta_dot: rad/sec
  note: Shortcuts
  note: BETA
  note: Input Variables
  note: ALPHA
  note: TAS
  tas : Inport
  beta : Inport  Port=2
  U : Inport  Port=3
  V : Inport  Port=4
  W : Inport  Port=5
  Udot : Inport  Port=6
  Vdot : Inport  Port=7
  Wdot : Inport  Port=8
  Cos : Trigonometry  Operator=cos
  Divide : Product  Inputs=*/
  Divide1 : Product  Inputs=*/
  Divide2 : Product  Inputs=**/
  Product{,1..6} (7 alike) : Product
  Square{,1..3} (4 alike) : Math  Operator=square  SignedPower=on  SaturateOnIntegerOverflow=on
  Sum : Sum  Inputs=+++
  Sum1 : Sum  Inputs=|-+
  Sum2 : Sum
  Sum3 : Sum  Inputs=|+-
  Sum4 : Sum
  tas_dot : Outport  VectorParamsAs1DForOutWhenUnconnected=off
  alpha_dot : Outport  Port=2  VectorParamsAs1DForOutWhenUnconnected=off
  beta_dot : Outport  Port=3  VectorParamsAs1DForOutWhenUnconnected=off
  wires:
  beta/1 -> [beta]
  tas/1 -> [tas]
  U/1 -> [U]
  V/1 -> [V]
  W/1 -> [W]
  Udot/1 -> [Udot]
  Vdot/1 -> [Vdot]
  Wdot/1 -> [Wdot]
  [beta] -> Cos/1
  Cos/1 -> [cbet]
  [U] -> Product/1
  [Wdot] -> Product2/2
  [W] -> Product2/1
  [Vdot] -> Product1/2
  [V] -> Product1/1
  [Udot] -> Product/2
  Product1/1 -> Sum/2
  Product/1 -> Sum/1
  Product2/1 -> Sum/3
  [tas] -> Divide/2
  Sum/1 -> Divide/1
  Square1/1 -> Sum2/2
  [W] -> Product3/1
  Divide1/1 -> alpha_dot/1
  Square/1 -> Sum2/1
  Product4/1 -> Sum1/2
  Sum1/1 -> Divide1/1
  [W] -> Square1/1
  Sum2/1 -> Divide1/2
  [U] -> Product4/1
  [Wdot] -> Product4/2
  [U] -> Square/1
  Product3/1 -> Sum1/1
  [Udot] -> Product3/2
  Divide/1 -> tas_dot/1, [tas_dot]
  Product6/1 -> Sum3/2
  Square2/1 -> Sum4/1
  Square3/1 -> Sum4/2
  [W] -> Square3/1
  [U] -> Square2/1
  Divide2/1 -> beta_dot/1
  Sum4/1 -> Divide2/3
  [V] -> Product6/1
  Product5/1 -> Sum3/1
  [tas_dot] -> Product6/2
  [cbet] -> Divide2/2
  [tas] -> Product5/1
  [Vdot] -> Product5/2
  Sum3/1 -> Divide2/1

== system f16_hifi_euler_vTrim/F-16 HiFi Model/Equation of Motion/Derivative Equations/Power Rate/cmd If ==
  note: Input Variables
  note: If
  note: Else
  note: If Condition
  cmdPower : Inport
  Power : Inport  Port=2
  Action Port : ActionPort  ActionPortLabel=if(u1 >= 50)
  If : If  IfExpression=u1 >= 50
  Merge : Merge
  Merge1 : Merge
  power else : Subsystem  TreatAsAtomicUnit=on
  power if : Subsystem  TreatAsAtomicUnit=on
  T : Outport  VectorParamsAs1DForOutWhenUnconnected=off
  P2 : Outport  Port=2  VectorParamsAs1DForOutWhenUnconnected=off
  wires:
  cmdPower/1 -> [cmdPower]
  Power/1 -> [Power]
  [Power] -> If/1
  If/1 -> [if]
  If/2 -> [else]
  [if] -> power if/Action
  [else] -> power else/Action
  [cmdPower] -> power if/1(cmdPower)
  Merge/1 -> T/1
  Merge1/1 -> P2/1
  power if/1(T) -> Merge/1
  power else/2(P2) -> Merge1/2
  power else/1(T) -> Merge/2
  power if/2(P2) -> Merge1/1
  [Power] -> power else/1(Power)

== system f16_hifi_euler_vTrim/F-16 HiFi Model/Equation of Motion/Derivative Equations/Power Rate/cmd else ==
  note: If
  note: Else
  note: Input Variables
  note: If Condition
  cmdPower : Inport
  Power : Inport  Port=2
  Action Port : ActionPort  ActionPortLabel=else
  If : If  IfExpression=u1 >= 50
  If Action Subsystem : Subsystem  TreatAsAtomicUnit=on
  Merge : Merge
  Merge1 : Merge
  power if : Subsystem  TreatAsAtomicUnit=on
  T : Outport  VectorParamsAs1DForOutWhenUnconnected=off
  P2 : Outport  Port=2  VectorParamsAs1DForOutWhenUnconnected=off
  wires:
  cmdPower/1 -> [cmdPower]
  Power/1 -> [Power]
  [Power] -> If/1
  If/1 -> [if]
  If/2 -> [else]
  [if] -> power if/Action
  [else] -> If Action Subsystem/Action
  [cmdPower] -> If Action Subsystem/1(cmdPower)
  [Power] -> If Action Subsystem/2(power)
  power if/2(P2) -> Merge1/1
  If Action Subsystem/1(T) -> Merge/2
  Merge1/1 -> P2/1
  If Action Subsystem/2(P2) -> Merge1/2
  power if/1(T) -> Merge/1
  Merge/1 -> T/1

== system f16_hifi_euler_vTrim/F-16 HiFi Model/Equation of Motion/Derivative Equations/Power Rate/cmd If/power else ==
  Power : Inport
  Action Port : ActionPort  ActionPortLabel=else
  Constant : Constant  Value=60
  RTAU : Subsystem
  Sum : Sum  Inputs=+-|
  T : Outport  VectorParamsAs1DForOutWhenUnconnected=off
  P2 : Outport  Port=2  VectorParamsAs1DForOutWhenUnconnected=off
  wires:
  Power/1 -> Sum/2
  RTAU/1(T) -> T/1
  Constant/1 -> Sum/1, P2/1
  Sum/1 -> RTAU/1(DP)

== system f16_hifi_euler_vTrim/F-16 HiFi Model/Equation of Motion/Derivative Equations/Power Rate/cmd If/power if ==
  cmdPower : Inport
  Action Port : ActionPort  ActionPortLabel=if(u1 >= 50)
  Constant : Constant  Value=5
  T : Outport  VectorParamsAs1DForOutWhenUnconnected=off
  P2 : Outport  Port=2  VectorParamsAs1DForOutWhenUnconnected=off
  wires:
  cmdPower/1 -> P2/1
  Constant/1 -> T/1

== system f16_hifi_euler_vTrim/F-16 HiFi Model/Equation of Motion/Derivative Equations/Power Rate/cmd else/If Action Subsystem ==
  cmdPower : Inport
  power : Inport  Port=2
  Action Port : ActionPort  ActionPortLabel=else
  RTAU : Subsystem
  Sum : Sum  Inputs=+-|
  T : Outport  VectorParamsAs1DForOutWhenUnconnected=off
  P2 : Outport  Port=2  VectorParamsAs1DForOutWhenUnconnected=off
  wires:
  power/1 -> Sum/2
  cmdPower/1 -> Sum/1, P2/1
  RTAU/1(T) -> T/1
  Sum/1 -> RTAU/1(DP)

== system f16_hifi_euler_vTrim/F-16 HiFi Model/Equation of Motion/Derivative Equations/Power Rate/cmd else/power if ==
  Action Port : ActionPort  ActionPortLabel=if(u1 >= 50)
  Constant : Constant  Value=5
  Constant1 : Constant  Value=40
  T : Outport  VectorParamsAs1DForOutWhenUnconnected=off
  P2 : Outport  Port=2  VectorParamsAs1DForOutWhenUnconnected=off
  wires:
  Constant/1 -> T/1
  Constant1/1 -> P2/1

== system f16_hifi_euler_vTrim/F-16 HiFi Model/Equation of Motion/Derivative Equations/Power Rate/cmd If/power else/RTAU ==
  DP : Inport
  If : If  IfExpression=u1 <= 25  ElseIfExpressions=u1 >= 50
  If Action Subsystem : Subsystem  TreatAsAtomicUnit=on
  If Action Subsystem1 : Subsystem  TreatAsAtomicUnit=on
  If Action Subsystem2 : Subsystem  TreatAsAtomicUnit=on
  Merge : Merge  Inputs=3
  T : Outport  VectorParamsAs1DForOutWhenUnconnected=off
  wires:
  DP/1 -> If Action Subsystem2/1(DP), If/1
  If/2 -> If Action Subsystem1/Action
  If/1 -> If Action Subsystem/Action
  If/3 -> If Action Subsystem2/Action
  If Action Subsystem/1(T) -> Merge/1
  If Action Subsystem1/1(T) -> Merge/2
  If Action Subsystem2/1(T) -> Merge/3
  Merge/1 -> T/1

== system f16_hifi_euler_vTrim/F-16 HiFi Model/Equation of Motion/Derivative Equations/Power Rate/cmd else/If Action Subsystem/RTAU ==
  DP : Inport
  If : If  IfExpression=u1 <= 25  ElseIfExpressions=u1 >= 50
  If Action Subsystem : Subsystem  TreatAsAtomicUnit=on
  If Action Subsystem1 : Subsystem  TreatAsAtomicUnit=on
  If Action Subsystem2 : Subsystem  TreatAsAtomicUnit=on
  Merge : Merge  Inputs=3
  T : Outport  VectorParamsAs1DForOutWhenUnconnected=off
  wires:
  Merge/1 -> T/1
  If Action Subsystem2/1(T) -> Merge/3
  If Action Subsystem1/1(T) -> Merge/2
  If Action Subsystem/1(T) -> Merge/1
  If/3 -> If Action Subsystem2/Action
  If/1 -> If Action Subsystem/Action
  If/2 -> If Action Subsystem1/Action
  DP/1 -> If/1, If Action Subsystem2/1(DP)

== system f16_hifi_euler_vTrim/F-16 HiFi Model/Equation of Motion/Derivative Equations/Power Rate/cmd If/power else/RTAU/If Action Subsystem ==
  Action Port : ActionPort  ActionPortLabel=if(u1 <= 25)
  Constant : Constant
  T : Outport  VectorParamsAs1DForOutWhenUnconnected=off
  wires:
  Constant/1 -> T/1

== system f16_hifi_euler_vTrim/F-16 HiFi Model/Equation of Motion/Derivative Equations/Power Rate/cmd If/power else/RTAU/If Action Subsystem1 ==
  Action Port : ActionPort  ActionPortLabel=elseif(u1 >= 50)
  Constant : Constant  Value=0.1
  T : Outport  VectorParamsAs1DForOutWhenUnconnected=off
  wires:
  Constant/1 -> T/1

== system f16_hifi_euler_vTrim/F-16 HiFi Model/Equation of Motion/Derivative Equations/Power Rate/cmd If/power else/RTAU/If Action Subsystem2 ==
  DP : Inport
  Action Port : ActionPort  ActionPortLabel=else
  Constant : Constant  Value=1.9
  Gain : Gain  Gain=0.036
  Sum : Sum  Inputs=|-+
  T : Outport  VectorParamsAs1DForOutWhenUnconnected=off
  wires:
  DP/1 -> Gain/1
  Gain/1 -> Sum/1
  Sum/1 -> T/1
  Constant/1 -> Sum/2

== system f16_hifi_euler_vTrim/F-16 HiFi Model/Equation of Motion/Derivative Equations/Power Rate/cmd else/If Action Subsystem/RTAU/If Action Subsystem ==
  Action Port : ActionPort  ActionPortLabel=if(u1 <= 25)
  Constant : Constant
  T : Outport  VectorParamsAs1DForOutWhenUnconnected=off
  wires:
  Constant/1 -> T/1

== system f16_hifi_euler_vTrim/F-16 HiFi Model/Equation of Motion/Derivative Equations/Power Rate/cmd else/If Action Subsystem/RTAU/If Action Subsystem1 ==
  Action Port : ActionPort  ActionPortLabel=elseif(u1 >= 50)
  Constant : Constant  Value=0.1
  T : Outport  VectorParamsAs1DForOutWhenUnconnected=off
  wires:
  Constant/1 -> T/1

== system f16_hifi_euler_vTrim/F-16 HiFi Model/Equation of Motion/Derivative Equations/Power Rate/cmd else/If Action Subsystem/RTAU/If Action Subsystem2 ==
  DP : Inport
  Action Port : ActionPort  ActionPortLabel=else
  Constant : Constant  Value=1.9
  Gain : Gain  Gain=0.036
  Sum : Sum  Inputs=|-+
  T : Outport  VectorParamsAs1DForOutWhenUnconnected=off
  wires:
  Constant/1 -> Sum/2
  Sum/1 -> T/1
  Gain/1 -> Sum/1
  DP/1 -> Gain/1
